simulink library "vmc"  (R2021b)
settings: Solver=VariableStepAuto  StartTime=0.0  StopTime=10.0  RelTol=1e-3
undefined symbols (not defined in the file or in its folder): AVMC_ACCDeltaTqIGain4OVRD_X_kph, AVMC_ACCDeltaTqIGain4OVRD_Y_mps2, AVMC_ACCDeltaTqIGain_X_kph, AVMC_ACCDeltaTqIGain_Y_mps2, AVMC_ACCDeltaTqPGain_X_kph, AVMC_ACCDeltaTqPGain_Y_kph, AVMC_ACCLongSteadyCtrl_X_kph, AVMC_ADSPosGFBDeltaTq_X_kph, AVMC_ADSPosGFBDeltaTq_Y_mps2, AVMC_AggressJerkPCT4AT_X_kph, AVMC_AggressJerkPCT_X_kph, AVMC_AggressLimitPCT4AT_X_kph, AVMC_AggressLimitPCT_X_kph, AVMC_CCLongSteadyCtrl_X_kph, AVMC_DISCDeltaTqIGain_X_kph, AVMC_DISCDeltaTqIGain_Y_mps2, AVMC_DISCDeltaTqPGain_X_kph, AVMC_DISCDeltaTqPGain_Y_kph, AVMC_ESCRegenOut_X_kph, AVMC_ESCRegenOut_Y_Deg, AVMC_ESCRegenOutEnSpd_X_Deg, AVMC_ISOAccLimit_X_mps, AVMC_ISODecLimit_X_mps, AVMC_ISOJerk_X_mps, AVMC_LatESCRegenOut_X_kph, AVMC_LatESCRegenOut_Y_Deg, AVMC_LongAccDeadZone_X_kph, AVMC_LongAccFiltTsforP2_X_Gps, AVMC_MCPresBaseTq_X_bar, AVMC_MSALongSteadyCtrl_X_kph, AVMC_MSAPedalOvrd_X_kph, AVMC_MSASpdBand_X_kph, AVMC_MSATqDownEndTq_X_kph, AVMC_MSATqDownTime_X_kph, AVMC_OPDDisSlideRate_X_Deg, AVMC_OVRD2ActSR2FCMCMD_X_mps2, AVMC_PedalTqRWhlRatio_X_Nm, AVMC_PedalTqRWhlRatio_Y_gps, AVMC_PedalTqRWhlSlipGain_X_rat, AVMC_PedalTqRWhlSlipGain_Y_kph, AVMC_PedalTqRWhSTRGGain_X_deg, AVMC_PedalTqRWhSTRGGain_Y_kph, AVMC_RDCDetectTime_X_kph, AVMC_RDCDetectTime_Y_pct, AVMC_RDCEnSlideRate_X_Deg, AVMC_RearWhlTqRatio_X_Nm, AVMC_RearWhlTqRatio_Y_gps, AVMC_RearWhlTqSlipGain_X_rat, AVMC_RearWhlTqSlipGain_Y_kph, AVMC_RearWhlTqSTRGGain_X_deg, AVMC_RearWhlTqSTRGGain_Y_kph, AVMC_ReqBrkJoinDecSR_X_mps2, AVMC_SoftJerkPCT_X_kph, AVMC_SoftLimitPCT_X_kph, AVMC_StESCYaw_X_kph, AVMC_StESCYaw_Y_Deg, AVMC_StESCYawCom_X_kph, AVMC_StESCYawCom_Y_Gps, AVMC_TMSpdBaseTq_X_rpm, AVMC_VehHoldDecCtrlTime2_X_kph ... (+411)
libraries: hcu_lib x108, simulink x82, tqr x1, simulink_extras x1
(part 7 of 14)

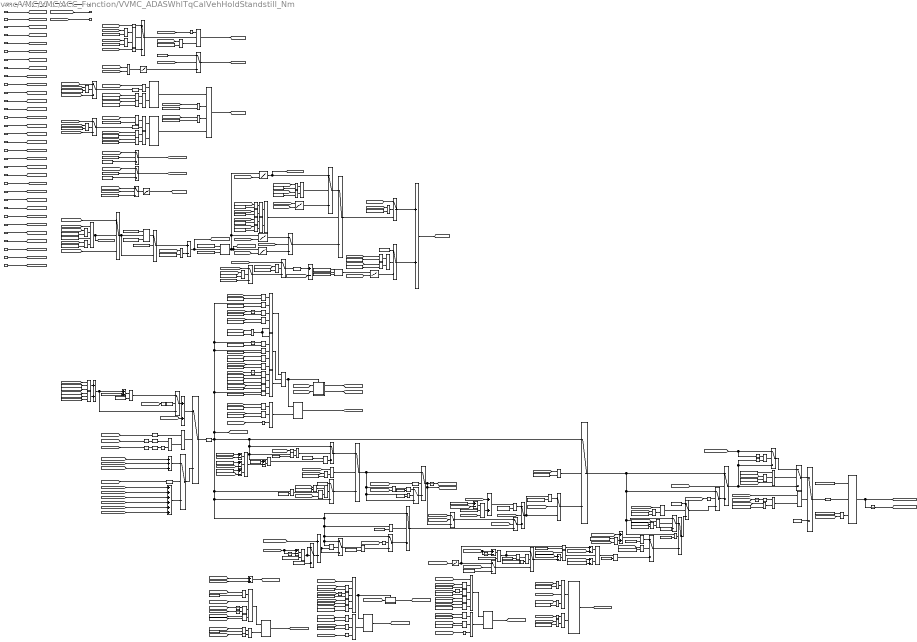
== system vmc/VMC/VMC/ACC_Function/VVMC_ADASWhlTqCalVehHoldStandstill_Nm ==
  note: Deceleration REGEN Torque Control
  note: Deceleration REGEN Torque Control Judgement
  note: Deceleration Torque Control
  note: Deceleration Positive Torque Control
  VVMC_LongAcc_Gps : Inport
  VVMC_ActACCRequiredAccel_mps2 : Inport  Port=2
  VINP_VehSpeed_kph : Inport  Port=3
  VVMC_ADASActive_flg : Inport  Port=4
  VTQD_CoordWhlTqDemFr_Nm : Inport  Port=5
  VTQD_CoordWhlTqDemRr_Nm : Inport  Port=6
  VVMC_ACCPedalOvrd_flg : Inport  Port=7
  VVMC_FeatSetSpdForCalcu_kph : Inport  Port=8
  VVMC_FeatArbitrFinal_enum : Inport  Port=9
  VINP_FrTMSpd_rpm : Inport  Port=10
  VINP_RrTMSpd_rpm : Inport  Port=11
  VINP_MCPressure_bar : Inport  Port=12
  VINP_ESCADASSta_enum : Inport  Port=13
  VVMC_FeatReqSpd_kph : Inport  Port=14
  VVMC_MeterIndSpeedForCalcu_kph : Inport  Port=15
  VTQD_SWC2ResUpSta_flg : Inport  Port=16
  VINP_FrntAxlTrqReqBrk_Nm : Inport  Port=17
  VINP_RearAxlTrqReqBrk_Nm : Inport  Port=18
  VTQR_RrTMTqReq_Nm : Inport  Port=19
  VVMC_ACCVehHoldReqRaw_flg : Inport  Port=20
  VVMC_EstSlope_Deg : Inport  Port=21
  VINP_TargetType_enum : Inport  Port=22
  VVMC_SafetyCtrl_flg : Inport  Port=23
  VTQR_FrTMTqReq_Nm : Inport  Port=24
  task_time_s : Inport  Port=25
  VVMC_TotalAvailBrkRgnTq_Nm : Inport  Port=26
  VVMC_AccelTurnHold_flg : Inport  Port=27
  VVMC_ADASACCSta_enum : Inport  Port=28
  VTQD_CreepBaseTqD_Nm : Inport  Port=29
  VVMC_OVRD2ActRampActive_flg : Inport  Port=30
  VINP_ACCRequiredAccel_mps2 : Inport  Port=31
  VTQD_SWC1ResUpSta_flg : Inport  Port=32
  VINP_SWCType_enum : Inport  Port=33
  " 1" : Constant  Value=ENUM_SWCTYPE_SWC2
  " 2" : Constant  Value=ENUM_SWCTYPE_SWC2
  AND{,1,4,7..8,10..11,13,17..18,20,29} (12 alike) : Logic  AllPortsSameDT=off  OutDataTypeStr=boolean
  AND12 : Logic  Inputs=3  AllPortsSameDT=off  OutDataTypeStr=boolean
  AND14 : Logic  Operator=OR  AllPortsSameDT=off  OutDataTypeStr=boolean
  AND19 : Logic  Operator=OR  AllPortsSameDT=off  OutDataTypeStr=boolean
  AND2 : Logic  Inputs=3  AllPortsSameDT=off  OutDataTypeStr=boolean
  AND3 : Logic  Inputs=4  AllPortsSameDT=off  OutDataTypeStr=boolean
  AND5 : Logic  Inputs=4  AllPortsSameDT=off  OutDataTypeStr=boolean
  AND6 : Logic  Inputs=3  AllPortsSameDT=off  OutDataTypeStr=boolean
  AND9 : Logic  Inputs=4  AllPortsSameDT=off  OutDataTypeStr=boolean
  Abs : Abs
  Abs1 : Abs
  Add{,3..4,7..8,10..12,14,16..17} (11 alike) : Sum  Inputs=+-
  Add1 : Sum  Inputs=++++++
  Add{2,5..6,13,15,19,21..23} (9 alike) : Sum
  Add9 : Sum  Inputs=+++
  Cast To Single2 : DataTypeConversion  OutDataTypeStr=single
  Cast To Single3 : DataTypeConversion  OutDataTypeStr=single
  Constant10 : Constant  Value=KVMC_ADASWhlTqUpperLim_Nm
  Constant100 : Constant  Value=KVMC_ZeroRgnTqSpdCtrlTime_s
  Constant{4,18..19,22,25,27,29,33,40,45,50..53,58,63..75,81..82,87,89..90,92..94,96,98..99,101..103,109,112,114,116..117,119..121,124..125,131..132,156,168} (56 alike) : Constant  Value=ZERO_FLOAT
  Constant104 : Constant  Value=KVMC_HoldAllowZeroTqGrade_deg
  Constant106 : Constant  Value=KVMC_VehHoldTqIncMinTq_Nm
  Constant107 : Constant  Value=KVMC_VehHoldTqIncMCP_bar
  Constant108 : Constant  Value=KVMC_VehHoldTqIncMCP_bar
  Constant11 : Constant  Value=KVMC_ADASWhlTqLowerLim_Nm
  Constant110 : Constant  Value=KVMC_NegReqEnSpd_kph
  Constant111 : Constant  Value=KVMC_VehHoldTqAlwaysIncSW_flg
  Constant12 : Constant  Value=KVMC_AccDevLowLim_mps2
  Constant122 : Constant  Value=KVMC_VehHoldDecSR_Nm
  Constant123 : Constant  Value=ENUM_FEATARBITRSTA_DISC
  Constant13 : Constant  Value=KVMC_AccDevUpLim_mps2
  Constant133 : Constant  Value=MINUSONE_FLOAT
  Constant138 : Constant  Value=KVMC_ReqAccelLimitSW_flg
  Constant139 : Constant  Value=KVMC_MaxReqAccel_mps2
  Constant14 : Constant  Value=KVMC_ACCSpdDevUpLim_kph
  Constant140 : Constant  Value=KVMC_MinReqAccel_mps2
  Constant15 : Constant  Value=KVMC_ACCSpdDevLowLim_kph
  Constant16 : Constant  Value=ENUM_FEATARBITRSTA_ACC
  Constant166 : Constant  Value=ENUM_ESCADASSTA_VEHASTANDSTILL
  Constant167 : Constant  Value=KVMC_StandstillTqRamp2ZeroSlope_Nmps
  Constant17 : Constant  Value=ENUM_ADASACCSTA_ACTIVE
  Constant{2,7..8,20} (4 alike) : Constant  Value=KVMC_HillUpResetTMSpd_rpm
  Constant21 : Constant  Value=ENUM_FEATARBITRSTA_DISC
  Constant23 : Constant  Value=KVMC_OVRDResSmoothTest_SW
  Constant24 : Constant  Value=KVMC_OVRD2ActRgnTarget_Nm
  Constant26 : Constant  Value=KVMC_AddBRegen2ACCLoop_flg
  Constant3 : Constant  Value=ENUM_ESCADASSTA_VEHASTANDSTILL
  Constant30 : Constant  Value=KVMC_TqSafetyCtrl_flg
  Constant31 : Constant  Value=KVMC_ACCResUpEnAccCMD_mps2
  Constant32 : Constant  Value=KVMC_TqMCPRelFactorHold_Nm
  Constant{6,36..37,62,77,80,88,97} (8 alike) : Constant  Value=KVMC_CutOffNegTqSpd_kph
  Constant38 : Constant  Value=KTQR_FrTMGearEff_c
  Constant{41,44,47..48,78..79,91} (7 alike) : Constant  Value=KVMC_ZeroRgnTqSpd_kph
  Constant42 : Constant  Value=KTQD_FrTMTotalGearRatio_gain
  Constant5 : Constant  Value=KVMC_AddBRegen2ACCLoop_flg
  Constant54 : Constant  Value=KVMC_NegReqSwEnSpd_kph
  Constant55 : Constant  Value=KVMC_NegReqSwEnSlope_Deg
  Constant56 : Constant  Value=KVMC_ACCResUpEnGrade_Deg
  Constant57 : Constant  Value=ENUM_TARGETTYPE_NONE
  Constant59 : Constant  Value=KVMC_TqMCPRelFactor_Nm
  Constant60 : Constant  Value=ENUM_FEATARBITRSTA_ACC
  Constant61 : Constant  Value=ENUM_FEATARBITRSTA_ACC
  Constant84 : Constant  Value=KTQD_RrTMTotalGearRatio_gain
  Constant85 : Constant  Value=KTQR_RrTMGearEff_c
  Constant86 : Constant  Value=KVMC_OVRDResTqDec4Smooth_Nm
  Constant9 : Constant  Value=KVMC_GravityValue_mps2
  Data Type Conversion1 : DataTypeConversion  OutDataTypeStr=single
  Detect Change : simulink/Logic and Bit Operations/Detect Change  vinit=0  OutDataTypeStr=boolean
  Detect Decrease1 : simulink/Logic and Bit Operations/Detect Decrease  vinit=0.0  OutDataTypeStr=boolean
  Detect Decrease2 : simulink/Logic and Bit Operations/Detect Decrease  vinit=0.0  OutDataTypeStr=boolean
  Detect Decrease3 : simulink/Logic and Bit Operations/Detect Decrease  vinit=0.0  OutDataTypeStr=boolean
  Detect Increase{1..4} (4 alike) : simulink/Logic and Bit Operations/Detect Increase  vinit=0.0  OutDataTypeStr=boolean
  Divide : Product  Inputs=*/*
  Divide1 : Product  Inputs=***
  Divide{2,4,7..8} (4 alike) : Product  Inputs=**
  Divide3 : Product  Inputs=*/*
  Divide5 : Product  Inputs=***
  Equal : RelationalOperator  Operator===  OutDataTypeStr=boolean  RndMeth=Simplest
  Equal1 : RelationalOperator  Operator=<=  OutDataTypeStr=boolean  RndMeth=Simplest
  Equal10 : RelationalOperator  Operator===  OutDataTypeStr=boolean  RndMeth=Simplest
  Equal{4,6,8,11} (4 alike) : RelationalOperator  Operator=<  OutDataTypeStr=boolean  RndMeth=Simplest
  Equal12 : RelationalOperator  Operator=>  OutDataTypeStr=boolean  RndMeth=Simplest
  Equal2 : RelationalOperator  Operator=~=  OutDataTypeStr=boolean  RndMeth=Simplest
  Equal3 : RelationalOperator  OutDataTypeStr=boolean  RndMeth=Simplest
  Equal5 : RelationalOperator  OutDataTypeStr=boolean  RndMeth=Simplest
  Equal7 : RelationalOperator  Operator=>  OutDataTypeStr=boolean  RndMeth=Simplest
  Equal9 : RelationalOperator  Operator=>  OutDataTypeStr=boolean  RndMeth=Simplest
  InitialCondition: 1 : UnitDelay  SampleTime=-1  HasFrameUpgradeWarning=on
  Logical Operator : Logic  Inputs=4  AllPortsSameDT=off  OutDataTypeStr=boolean
  Logical Operator1 : Logic  Operator=OR  AllPortsSameDT=off  OutDataTypeStr=boolean
  Logical Operator{2,4,6,8} (4 alike) : Logic  Inputs=5  AllPortsSameDT=off  OutDataTypeStr=boolean
  Logical Operator3 : Logic  Operator=OR  Inputs=3  AllPortsSameDT=off  OutDataTypeStr=boolean
  Logical Operator5 : Logic  AllPortsSameDT=off  OutDataTypeStr=boolean
  Logical Operator7 : Logic  Operator=OR  Inputs=3  AllPortsSameDT=off  OutDataTypeStr=boolean
  Logical Operator9 : Logic  Operator=OR  Inputs=3  AllPortsSameDT=off  OutDataTypeStr=boolean
  MVMC_ACCDeltaTqIGain4OVRD_Z_Nm : Lookup_n-D  BreakpointsForDimension1=AVMC_ACCDeltaTqIGain4OVRD_Y_mps2  BreakpointsForDimension2=AVMC_ACCDeltaTqIGain4OVRD_X_kph  Table=MVMC_ACCDeltaTqIGain4OVRD_Z_Nm  InternalRulePriority=Speed  RndMeth=Simplest  InputSameDT=on
      settings: InputPortMap=u0,u1
  MVMC_ACCDeltaTqIGain_Z_Nm : Lookup_n-D  BreakpointsForDimension1=AVMC_ACCDeltaTqIGain_Y_mps2  BreakpointsForDimension2=AVMC_ACCDeltaTqIGain_X_kph  Table=MVMC_ACCDeltaTqIGain_Z_Nm  InternalRulePriority=Speed  RndMeth=Simplest  InputSameDT=on
      settings: InputPortMap=u0,u1
  MVMC_ACCDeltaTqPGain_Z_Nm1 : Lookup_n-D  BreakpointsForDimension1=AVMC_ACCDeltaTqPGain_Y_kph  BreakpointsForDimension2=AVMC_ACCDeltaTqPGain_X_kph  Table=MVMC_ACCDeltaTqPGain_Z_Nm  InternalRulePriority=Speed  RndMeth=Simplest  InputSameDT=on
      settings: InputPortMap=u0,u1
  MVMC_ADSPosGFBDeltaTq_Z_Nm1 : Lookup_n-D  BreakpointsForDimension1=AVMC_ADSPosGFBDeltaTq_Y_mps2  BreakpointsForDimension2=AVMC_ADSPosGFBDeltaTq_X_kph  Table=MVMC_ADSPosGFBDeltaTq_Z_Nm  InternalRulePriority=Speed  RndMeth=Simplest  InputSameDT=on
      settings: InputPortMap=u0,u1
  MVMC_DISCDeltaTqIGain_Z_Nm : Lookup_n-D  BreakpointsForDimension1=AVMC_DISCDeltaTqIGain_Y_mps2  BreakpointsForDimension2=AVMC_DISCDeltaTqIGain_X_kph  Table=MVMC_DISCDeltaTqIGain_Z_Nm  InternalRulePriority=Speed  RndMeth=Simplest  InputSameDT=on
      settings: InputPortMap=u0,u1
  MVMC_MCPresBaseTq_Y_Nm : Lookup_n-D  NumberOfTableDimensions=1  BreakpointsForDimension1=AVMC_MCPresBaseTq_X_bar  Table=MVMC_MCPresBaseTq_Y_Nm  InternalRulePriority=Speed  RndMeth=Simplest  InputSameDT=on
  MVMC_TMSpdBaseTq_Y_Nm : Lookup_n-D  NumberOfTableDimensions=1  BreakpointsForDimension1=AVMC_TMSpdBaseTq_X_rpm  Table=MVMC_TMSpdBaseTq_Y_Nm  InternalRulePriority=Speed  RndMeth=Simplest  InputSameDT=on
  MVMC_VehHoldTqIncGain_Y_Nm : Lookup_n-D  NumberOfTableDimensions=1  BreakpointsForDimension1=AVMC_VehHoldTqIncGain_X_deg  Table=MVMC_VehHoldTqIncGain_Y_Nm  InternalRulePriority=Speed  RndMeth=Simplest  InputSameDT=on
  Max{,1,4..6,8} (6 alike) : MinMax  Function=max  Inputs=2
  Max2 : MinMax  Inputs=2
  Max3 : MinMax  Inputs=2
  Max9 : MinMax  Inputs=2
  Min : MinMax  Inputs=2
  Min1 : MinMax  Inputs=2
  Min2 : MinMax  Function=max  Inputs=2
  Min5 : MinMax  Function=max  Inputs=2
  NOT{,1..10,13} (12 alike) : Logic  Operator=NOT  AllPortsSameDT=off  OutDataTypeStr=boolean
  OR{,1,4,6..8} (6 alike) : Logic  Operator=OR  AllPortsSameDT=off  OutDataTypeStr=boolean
  OR3 : Logic  Operator=OR  Inputs=3  AllPortsSameDT=off  OutDataTypeStr=boolean
  OR5 : Logic  AllPortsSameDT=off  OutDataTypeStr=boolean
  Product1 : Product
  Relational Operator{,2..4,7,13,16,27,32..33,38,44,47,58..59,61} (16 alike) : RelationalOperator  Operator=>  OutDataTypeStr=boolean  RndMeth=Simplest
  Relational Operator{1,18,20,34,40,51} (6 alike) : RelationalOperator  Operator=<=  OutDataTypeStr=boolean  RndMeth=Simplest
  Relational Operator{8,10,12,24..25,29,36..37,39,42..43,48,53} (13 alike) : RelationalOperator  OutDataTypeStr=boolean  RndMeth=Simplest
  Relational Operator{9,11,14..15,21..23,26,28,30..31,35,41,45..46,49..50,52,54} (19 alike) : RelationalOperator  Operator=<  OutDataTypeStr=boolean  RndMeth=Simplest
  Relational Operator{5..6,17,19,55..57,73} (8 alike) : RelationalOperator  Operator===  OutDataTypeStr=boolean  RndMeth=Simplest
  Relay : Relay  OnSwitchValue=KVMC_ACCTq2ZeroEnMCPress2_bar  OffSwitchValue=KVMC_ACCTq2ZeroDisMCPress2_bar  OutDataTypeStr=boolean
  Relay1 : Relay  OnSwitchValue=KVMC_ACCTq2ZeroEnMCPress_bar  OffSwitchValue=KVMC_ACCTq2ZeroDisMCPress_bar  OutDataTypeStr=boolean
  SR_Latch{,1..6} (7 alike) : hcu_lib/Basic_Blocks/SR_Latch
  Saturation Dynamic{1..5} (5 alike) : simulink/Discontinuities/Saturation Dynamic  OutMin=[]  OutMax=[]  OutDataTypeStr=Inherit: Same as second input  OutDataType=fixdt(1, 16)  OutScaling=2^-10  DoSatur=off
  Switch{,1..34,36..37,39..41} (40 alike) : Switch  Criteria=u2 > Threshold
  Triggered Subsystem1 : Subsystem  TreatAsAtomicUnit=on
  Triggered Subsystem4 : Subsystem  TreatAsAtomicUnit=on
  Unit Delay{,1..13} (14 alike) : UnitDelay  SampleTime=-1  HasFrameUpgradeWarning=on
  u2 > 0 : Switch  Criteria=u2 > Threshold
  u2 > 0 (1) : Switch  Criteria=u2 > Threshold
  u2 > 0 (3) : Switch  Criteria=u2 > Threshold
  u2 > 0 (4) : Switch  Criteria=u2 > Threshold
  VVMC_ADASWhlTqCal_Nm : Outport
  VVMC_ADASNegReq_flg : Outport  Port=2
  VVMC_ACCLowSpdTqCtrl_flg : Outport  Port=3
  wires:
  VVMC_FeatReqSpd_kph/1 -> [VVMC_FeatReqSpd_kph]
  [VINP_RrTMSpd_rpm] -> Relational Operator2/1
  [VVMC_ACCVehHoldReqRaw_flg] -> AND4/1
  MVMC_MCPresBaseTq_Y_Nm/1 -> [VVMC_MCPresBaseTq_Nm]  "VVMC_MCPresBaseTq_Nm"
  Switch1/1 -> MVMC_MCPresBaseTq_Y_Nm/1
  [VINP_MCPressure_bar] -> Switch1/1
  Relational Operator/1 -> OR/1
  Equal/1 -> AND1/1
  OR/1 -> SR_Latch/2
  [VINP_FrTMSpd_rpm] -> Relational Operator/1
  [VINP_ESCADASSta_enum] -> Equal/1
  [VINP_RrTMSpd_rpm] -> Relational Operator4/1
  AND1/1 -> SR_Latch1/1
  Relational Operator2/1 -> OR/2
  OR1/1 -> SR_Latch1/2
  Constant19/1 -> Switch1/3
  Constant8/1 -> Relational Operator3/2
  Relational Operator4/1 -> OR1/2
  [VVMC_MCPreBaseTqEn_flg] -> Switch1/2
  [VINP_FrTMSpd_rpm] -> Relational Operator3/1
  Constant7/1 -> Relational Operator4/2
  Constant2/1 -> Relational Operator2/2
  Detect Increase3/1 -> AND1/2
  SR_Latch/1 -> AND3/1  "VVMC_HillUpHoldReqEn_flg"
  AND3/1 -> [VVMC_MCPreBaseTqEn_flg]  "VVMC_MCPreBaseTqEn_flg"
  SR_Latch1/1 -> AND3/4  "VVMC_HillUpESCStaEn_flg"
  Constant3/1 -> Equal/2
  Constant20/1 -> Relational Operator/2
  Relational Operator3/1 -> OR1/1
  VINP_FrTMSpd_rpm/1 -> [VINP_FrTMSpd_rpm]
  VINP_RrTMSpd_rpm/1 -> [VINP_RrTMSpd_rpm]
  VINP_MCPressure_bar/1 -> [VINP_MCPressure_bar]
  VINP_ESCADASSta_enum/1 -> [VINP_ESCADASSta_enum]
  VVMC_FeatArbitrFinal_enum/1 -> [VVMC_FeatArbitrFinal_enum]
  VVMC_LongAcc_Gps/1 -> [VVMC_LongAcc_Gps]
  VVMC_ActACCRequiredAccel_mps2/1 -> [VVMC_ActACCRequiredAccel_mps2]
  VINP_VehSpeed_kph/1 -> [VINP_VehSpeed_kph]
  VVMC_ADASActive_flg/1 -> [VVMC_ADASActive_flg]
  [VVMC_ADASWhlTqCal_Nm] -> VVMC_ADASWhlTqCal_Nm/1
  VTQD_CoordWhlTqDemFr_Nm/1 -> [VTQD_CoordWhlTqDemFr_Nm]
  VTQD_CoordWhlTqDemRr_Nm/1 -> [VTQD_CoordWhlTqDemRr_Nm]
  VVMC_ACCPedalOvrd_flg/1 -> [VVMC_ACCPedalOvrd_flg]
  VVMC_FeatSetSpdForCalcu_kph/1 -> [VVMC_FeatSetSpdForCalcu_kph]
  VINP_RearAxlTrqReqBrk_Nm/1 -> [VINP_RearAxlTrqReqBrk_Nm]
  VINP_FrntAxlTrqReqBrk_Nm/1 -> [VINP_FrntAxlTrqReqBrk_Nm]
  VTQD_SWC2ResUpSta_flg/1 -> [VTQD_SWC2ResUpSta_flg]
  VVMC_MeterIndSpeedForCalcu_kph/1 -> [VVMC_MeterIndSpeedForCalcu_kph]
  Switch32/1 -> Detect Increase2/1
  AND4/1 -> SR_Latch/1
  [VVMC_ActACCRequiredAccel_mps2] -> Relational Operator7/1
  Constant31/1 -> Relational Operator7/2
  Switch2/1 -> Detect Increase3/1
  [VINP_FrntAxlTrqReqBrk_Nm] -> Switch3/1
  [VINP_RearAxlTrqReqBrk_Nm] -> Switch4/1
  Constant25/1 -> Switch3/3
  Constant27/1 -> Switch4/3
  Constant26/1 -> Switch4/2
  Switch4/1 -> [VVMC_RearAxlTrqReqBrk_Nm]  "VVMC_RearAxlTrqReqBrk_Nm"
  Switch3/1 -> [VVMC_FrntAxlTrqReqBrk_Nm]  "VVMC_FrntAxlTrqReqBrk_Nm"
  Constant5/1 -> Switch3/2
  [VVMC_ADASNegReq_flg] -> VVMC_ADASNegReq_flg/1
  VTQR_RrTMTqReq_Nm/1 -> [VTQR_RrTMTqReq_Nm]
  VVMC_ACCVehHoldReqRaw_flg/1 -> [VVMC_ACCVehHoldReqRaw_flg]
  [VVMC_EstSlope_Deg] -> Relational Operator16/1
  Relational Operator16/1 -> AND3/3
  Constant56/1 -> Relational Operator16/2
  VVMC_EstSlope_Deg/1 -> [VVMC_EstSlope_Deg]
  VINP_TargetType_enum/1 -> [VINP_TargetType_enum]
  VVMC_SafetyCtrl_flg/1 -> [VVMC_SafetyCtrl_flg]
  VTQR_FrTMTqReq_Nm/1 -> [VTQR_FrTMTqReq_Nm]
  [VVMC_ACCLowSpdTqCtrl_flg] -> VVMC_ACCLowSpdTqCtrl_flg/1
  task_time_s/1 -> [task_time_s]
  MVMC_TMSpdBaseTq_Y_Nm/1 -> Switch/3
  [VVMC_ACCVehHoldReqRaw_flg] -> Switch/2
  Relay/1 -> Switch13/1
  Switch13/1 -> AND2/2  "VVMC_ADASNegReqAct_flg"
  AND2/1 -> [VVMC_ADASNegReq_flg]  "VVMC_ADASNegReq_flg"
  [VINP_RrTMSpd_rpm] -> Min/2
  [VVMC_MCPreBaseTqEn_flg] -> NOT2/1
  Equal5/1 -> AND2/3
  [VINP_VehSpeed_kph] -> Equal5/1
  [VINP_FrTMSpd_rpm] -> Min/1
  Constant110/1 -> Equal5/2
  [VINP_MCPressure_bar] -> Relay/1
  [VINP_VehSpeed_kph] -> Equal1/1
  Equal3/1 -> AND10/2
  Relay1/1 -> Switch13/3
  Switch/1 -> [VVMC_TMSpdBaseTq_Nm]  "VVMC_TMSpdBaseTq_Nm"
  Constant54/1 -> Equal1/2
  [VINP_MCPressure_bar] -> Relay1/1
  AND10/1 -> Switch13/2
  Constant55/1 -> Equal3/2
  [VVMC_EstSlope_Deg] -> Equal3/1
  Equal1/1 -> AND10/1
  Min/1 -> MVMC_TMSpdBaseTq_Y_Nm/1
  NOT2/1 -> AND2/1
  Constant119/1 -> Switch/1
  Switch29/1 -> Switch22/3
  [VINP_VehSpeed_kph] -> Relational Operator21/1
  [VINP_VehSpeed_kph] -> Relational Operator20/1
  Relational Operator11/1 -> Logical Operator/2
  SR_Latch4/1 -> [VVMC_ZeroRgnTqSpdCtrl_flg]  "VVMC_ZeroRgnTqSpdCtrl_flg"
  Constant48/1 -> Add4/1
  Relational Operator31/1 -> Logical Operator4/1
  [VVMC_ActACCRequiredAccel_mps2] -> Relational Operator41/1
  Logical Operator2/1 -> OR3/2
  Constant93/1 -> Relational Operator42/2
  Relational Operator25/1 -> Logical Operator2/2
  Max1/1 -> Switch23/1
  Logical Operator/1 -> OR3/3
  [VVMC_LastADASWhlTqCal_Nm] -> Add12/1
  [VINP_VehSpeed_kph] -> Relational Operator8/1
  [VVMC_ADASActive_flg] -> NOT1/1
  Constant63/1 -> Min2/2
  Logical Operator3/1 -> SR_Latch6/2
  Constant29/1 -> Relational Operator10/2
  Relational Operator8/1 -> Logical Operator3/1
  Unit Delay/1 -> Relational Operator12/1
  [VVMC_TMSpdBaseTq_Nm] -> Add1/3
  Logical Operator1/1 -> Switch6/2
  Constant36/1 -> Relational Operator11/2
  NOT1/1 -> Logical Operator3/3
  [VINP_MCPressure_bar] -> Add11/1, Unit Delay5/1
  [VVMC_FrntAxlTrqReqBrk_Nm] -> Add1/5
  [VTQD_CoordWhlTqDemFr_Nm] -> Add9/1
  Divide2/1 -> Switch15/1, Switch15/2
  Constant92/1 -> Relational Operator41/2
  Constant84/1 -> Divide5/2
  Relational Operator15/1 -> Logical Operator/4
  [VVMC_ActACCRequiredAccel_mps2] -> Relational Operator10/1
  Constant114/1 -> Relational Operator49/2
  AND13/1 -> Switch21/2
  Constant69/1 -> Switch15/3
  Add14/1 -> Divide3/1
  Constant101/1 -> Max2/2
  Switch23/1 -> Switch17/3  "VVMC_ADASWhlTqCalNegCMD_Nm"
  Constant70/1 -> Relational Operator26/2
  [VVMC_MCPresBaseTq_Nm] -> Add1/4
  [VINP_VehSpeed_kph] -> Relational Operator44/1
  Switch10/1 -> Min2/1
  Constant64/1 -> Relational Operator22/2
  Min2/1 -> Switch16/3  "VVMC_ACCTqNegReq_Nm"
  [VTQR_RrTMTqReq_Nm] -> Divide5/1
  Triggered Subsystem1/2(Out2) -> [VVMC_ACCLowSpdCtrlEnSpd_kph]  "VVMC_ACCLowSpdCtrlEnSpd_kph"
  NOT9/1 -> Logical Operator9/3
  Switch6/1 -> Cast To Single2/1
  Logical Operator8/1 -> SR_Latch4/1, Triggered Subsystem4/Trigger
  Cast To Single2/1 -> Switch19/1, Relational Operator26/1, Switch16/1, Switch10/1, Relational Operator9/1, Switch21/3, Relational Operator49/1, Switch27/1, Max4/1, Relational Operator47/1, Switch17/1, [VVMC_OriADASWhlTq_Nm], Relational Operator30/1, Unit Delay3/1, Relational Operator23/1, Relational Operator15/1  "VVMC_OriADASWhlTq_Nm"
  Add11/1 -> Divide2/1
  Unit Delay7/1 -> [VVMC_LastACCLowSpdTq_Nm]
  Detect Increase1/1 -> Logical Operator1/1
  [VVMC_ZeroRgnTqSpdCtrl_flg] -> Switch24/2
  Add15/1 -> Max2/1  "VVMC_ADASWhlTqCalZeroRgnCtrl_Nm"
  Add5/1 -> Switch6/1
  Divide1/1 -> Add13/1
  Triggered Subsystem4/1(Out1) -> [VVMC_ZeroRgnTqSpdCtrlTq_Nm]  "VVMC_ZeroRgnTqSpdCtrlTq_Nm"
  Unit Delay9/1 -> Relational Operator42/1
  Detect Decrease2/1 -> Switch8/2
  Add13/1 -> Switch36/3, Add23/1
  [VVMC_LastADASWhlTqCal_Nm] -> Relational Operator45/1
  Relational Operator32/1 -> Logical Operator4/5, Logical Operator2/1
  [VVMC_LastADASWhlTqCal_Nm] -> Triggered Subsystem4/1(In1)
  Constant96/1 -> Relational Operator43/2
  [VINP_VehSpeed_kph] -> Relational Operator40/1
  Divide/1 -> Add/2
  Constant67/1 -> Relational Operator25/2
  Relational Operator44/1 -> Logical Operator9/1
  Relational Operator30/1 -> Logical Operator4/2
  Switch21/1 -> Switch12/3  "VVMC_ACCLowSpdTqEnSpdLo_Nm"
  [VVMC_ActACCRequiredAccel_mps2] -> Unit Delay6/1
  [VVMC_ActACCRequiredAccel_mps2] -> Relational Operator43/1
  Constant97/1 -> Relational Operator44/2
  [VVMC_ADASActive_flg] -> NOT9/1
  Add/1 -> Max4/2
  Relational Operator29/1 -> Logical Operator4/3
  Relational Operator45/1 -> Logical Operator8/2
  Constant98/1 -> Relational Operator45/2
  Constant6/1 -> Relational Operator8/2
  [VVMC_ActACCRequiredAccel_mps2] -> Unit Delay9/1
  Switch18/1 -> Switch24/3
  Add1/1 -> Switch8/3
  Constant100/1 -> Divide3/2
  Constant89/1 -> Max1/2
  [VVMC_RgnProhibited_flg] -> Switch23/2
  [VINP_VehSpeed_kph] -> Relational Operator31/1
  [task_time_s] -> Divide3/3
  Constant53/1 -> Switch21/1
  Max2/1 -> Switch24/1
  Constant99/1 -> Add14/1
  Relational Operator12/1 -> Logical Operator/1
  [VVMC_LastACCLowSpdTq_Nm] -> Max/2
  Switch12/1 -> Switch22/1, Switch29/3, Relational Operator50/1, Max/1
  Switch15/1 -> Add12/2
  Constant117/1 -> Max3/2
  Add9/1 -> Switch8/1
  [VVMC_ActACCRequiredAccel_mps2] -> Relational Operator24/1
  [VVMC_ACCLowSpdCtrlEnSpd_kph] -> Add4/2
  Min1/1 -> Switch27/3
  Relational Operator20/1 -> AND13/1
  Relational Operator47/1 -> AND8/2
  Max/1 -> Max3/1
  Relational Operator43/1 -> Logical Operator9/2
  Constant47/1 -> Add3/1
  [VVMC_ACCLowSpdTqCtrl_flg] -> Detect Increase4/1
  Constant4/1 -> Relational Operator24/2
  Unit Delay5/1 -> Add11/2
  Max3/1 -> Switch29/1
  Detect Increase4/1 -> Switch22/2
  Constant78/1 -> Relational Operator32/2
  Constant79/1 -> Relational Operator33/2
  [VINP_VehSpeed_kph] -> Relational Operator32/1
  [VVMC_ACCLowSpdCtrlEnSpd_kph] -> Relational Operator33/1
  [VVMC_ZeroRgnTqSpdCtrlTq_Nm] -> Add14/2
  Constant77/1 -> Relational Operator31/2
  Constant75/1 -> Relational Operator30/2
  Logical Operator4/1 -> OR3/1
  Constant73/1 -> Relational Operator29/2
  Relational Operator42/1 -> Logical Operator8/3
  Constant72/1 -> Relational Operator28/2
  [VVMC_ADASActive_flg] -> Detect Increase1/1
  Relational Operator28/1 -> Logical Operator4/4
  [VVMC_ActACCRequiredAccel_mps2] -> Relational Operator28/1
  [VVMC_RearAxlTrqReqBrk_Nm] -> Add1/6
  Constant40/1 -> Relational Operator14/2
  Relational Operator41/1 -> Logical Operator8/4
  Switch24/1 -> Max1/1, Switch23/3
  [VINP_VehSpeed_kph] -> Unit Delay/1
  [VINP_VehSpeed_kph] -> Triggered Subsystem1/2(In2)
  Unit Delay3/1 -> Relational Operator25/1
  Relational Operator26/1 -> Switch19/2
  AND14/1 -> AND13/2
  Constant38/1 -> Divide1/3
  Switch22/1 -> Unit Delay7/1, Switch20/3, [VVMC_ACCLowSpdTq_Nm]  "VVMC_ACCLowSpdTq_Nm"
  [VVMC_ACCLowSpdTqCtrl_flg] -> Logical Operator5/1
  OR3/1 -> SR_Latch6/1, Triggered Subsystem1/Trigger
  Relational Operator23/1 -> Logical Operator2/3
  [VVMC_ActACCRequiredAccel_mps2] -> Relational Operator22/1
  [VTQR_FrTMTqReq_Nm] -> Divide1/1
  Switch27/1 -> Switch12/1  "VVMC_ACCLowSpdTqEnSpdHi_Nm"
  Relational Operator21/1 -> Logical Operator2/4
  Constant62/1 -> Relational Operator21/2
  Relational Operator10/1 -> Logical Operator3/2
  Unit Delay6/1 -> Relational Operator29/1
  [VINP_VehSpeed_kph] -> Relational Operator11/1
  Add10/1 -> Divide/3
  Constant112/1 -> Relational Operator47/2
  Logical Operator5/1 -> Switch12/2
  AND/1 -> Logical Operator1/2
  Constant52/1 -> Min1/1
  Relational Operator9/1 -> Switch10/2
  Add12/1 -> Relational Operator9/2, Switch10/3  "VVMC_ACCTqRampOutByMCP_Nm"
  Add4/1 -> Divide/2
  [VVMC_LastADASWhlTqCal_Nm] -> Add15/1
  Add3/1 -> Divide/1
  [VVMC_ADASNegReq_flg] -> Detect Decrease2/1
  Divide5/1 -> Add13/2
  Relational Operator24/1 -> Switch17/2
  Constant85/1 -> Divide5/3
  Constant50/1 -> Add10/1
  Constant37/1 -> Relational Operator12/2
  [VVMC_ACCDeltaTq_Nm] -> Add9/3
  Relational Operator22/1 -> Logical Operator2/5
  Constant66/1 -> Relational Operator23/2
  Constant45/1 -> Relational Operator15/2
  Relational Operator40/1 -> Logical Operator8/5
  Constant42/1 -> Divide1/2
  [VVMC_ActACCRequiredAccel_mps2] -> Relational Operator14/1
  Relational Operator14/1 -> Logical Operator/3
  [VVMC_ACCDeltaTq_Nm] -> Add1/2
  [VVMC_LastADASWhlTqCal_Nm] -> Add1/1
  [VVMC_ACCLowSpdTqLimit_Nm] -> Add10/2
  Triggered Subsystem1/1(Out1) -> [VVMC_ACCLowSpdTqLimit_Nm]  "VVMC_ACCLowSpdTqLimit_Nm"
  Constant116/1 -> Relational Operator50/2
  Relational Operator33/1 -> Logical Operator5/2
  [VINP_VehSpeed_kph] -> Add3/2
  Constant51/1 -> Add/1
  [VVMC_ACCLowSpdTqCtrl_flg] -> Switch18/2
  [VTQD_CoordWhlTqDemRr_Nm] -> Add9/2
  SR_Latch6/1 -> [VVMC_ACCLowSpdTqCtrl_flg]  "VVMC_ACCLowSpdTqCtrl_flg"
  Constant91/1 -> Relational Operator40/2
  Constant41/1 -> Relational Operator20/2
  Divide3/1 -> Add15/2
  [VVMC_ACCDeltaTq_Nm] -> Add5/2
  Constant59/1 -> Divide2/2
  Relational Operator49/1 -> AND14/1
  AND8/1 -> Switch27/2
  NOT13/1 -> AND8/1
  [VVMC_ADASNegReq_flg] -> NOT13/1
  Constant12/1 -> Saturation Dynamic4/3
  Saturation Dynamic4/1 -> MVMC_DISCDeltaTqIGain_Z_Nm/1, MVMC_ACCDeltaTqIGain4OVRD_Z_Nm/1, [VVMC_ActAccDev_mps2], MVMC_ACCDeltaTqIGain_Z_Nm/1  "VVMC_ActAccDev_mps2"
  Switch33/1 -> Add6/1  "VVMC_ACCDeltaTqIGain_Nm"
  Saturation Dynamic5/1 -> MVMC_ACCDeltaTqPGain_Z_Nm1/1  "VVMC_ACCActSpdDev_kph"
  [VVMC_LongAcc_Gps] -> Product1/1
  Constant16/1 -> Relational Operator5/2
  [VVMC_FeatArbitrFinal_enum] -> Relational Operator6/1
  [VVMC_FeatArbitrFinal_enum] -> Relational Operator5/1
  [VVMC_FeatReqSpd_kph] -> u2 > 0 (1)/1
  Constant15/1 -> Saturation Dynamic5/3
  Equal2/1 -> AND11/1
  Product1/1 -> Add7/2
  Constant21/1 -> Relational Operator6/2
  Constant60/1 -> Relational Operator17/2
  u2 > 0/1 -> Data Type Conversion1/1
  u2 > 0 (1)/1 -> u2 > 0/3
  [VVMC_MeterIndSpeedForCalcu_kph] -> Add8/2
  [VVMC_LongAcc_Gps] -> Equal6/1
  AND17/1 -> AND19/1
  [VVMC_ActACCRequiredAccel_mps2] -> Equal7/1
  [VINP_VehSpeed_kph] -> MVMC_DISCDeltaTqIGain_Z_Nm/2
  Constant125/1 -> Equal7/2
  [VINP_TargetType_enum] -> Equal2/1
  MVMC_DISCDeltaTqIGain_Z_Nm/1 -> [VVMC_DISCDeltaTqIGain_Nm], Switch40/1  "VVMC_DISCDeltaTqIGain_Nm"
  Constant124/1 -> Equal6/2
  Data Type Conversion1/1 -> Add8/1
  Relational Operator5/1 -> u2 > 0/2
  Add6/1 -> [VVMC_ACCDeltaTq_Nm]  "VVMC_ACCDeltaTq_Nm"
  MVMC_ACCDeltaTqIGain_Z_Nm/1 -> Switch26/3  "VVMC_ACCDeltaTqIGainOri_Nm"
  Constant13/1 -> Saturation Dynamic4/1
  [VVMC_FeatArbitrFinal_enum] -> Relational Operator55/1
  Relational Operator55/1 -> Switch33/2
  Constant9/1 -> Product1/2
  [VINP_VehSpeed_kph] -> MVMC_ACCDeltaTqIGain_Z_Nm/2
  Equal6/1 -> AND17/1
  Add8/1 -> Saturation Dynamic5/2
  [VINP_VehSpeed_kph] -> MVMC_ACCDeltaTqPGain_Z_Nm1/2
  Add7/1 -> [VVMC_ACCDeltaAccel_mps2], Saturation Dynamic4/2  "VVMC_ACCDeltaAccel_mps2"
  Constant123/1 -> Relational Operator55/2
  Constant22/1 -> u2 > 0 (1)/3
  Constant14/1 -> Saturation Dynamic5/1
  Equal7/1 -> AND17/2
  AND11/1 -> Switch14/2
  Relational Operator6/1 -> u2 > 0 (1)/2
  [VVMC_FeatSetSpdForCalcu_kph] -> u2 > 0/1
  MVMC_ACCDeltaTqPGain_Z_Nm1/1 -> Switch14/3
  Relational Operator17/1 -> AND11/2
  [VVMC_FeatArbitrFinal_enum] -> Relational Operator17/1
  Constant57/1 -> Equal2/2
  Switch34/1 -> Switch33/3
  Constant58/1 -> Switch14/1
  Switch14/1 -> Add6/2  "VVMC_ACCDeltaTqPGain_Nm"
  AND19/1 -> Switch34/2
  Constant131/1 -> Equal8/2
  [VVMC_ActACCRequiredAccel_mps2] -> Equal8/1
  Equal8/1 -> AND20/1
  AND20/1 -> AND19/2
  Equal9/1 -> AND20/2
  [VVMC_ACCDeltaAccel_mps2] -> Equal9/1
  Constant132/1 -> Equal9/2
  Switch19/1 -> Switch18/3  "VVMC_ACCTqNegReqNotLowSpd_Nm"
  Detect Increase2/1 -> AND4/2
  Relational Operator7/1 -> AND3/2
  VVMC_TotalAvailBrkRgnTq_Nm/1 -> [VVMC_TotalAvailBrkRgnTq_Nm]
  VVMC_AccelTurnHold_flg/1 -> [VVMC_AccelTurnHold_flg]
  VVMC_ADASACCSta_enum/1 -> [VVMC_ADASACCSta_enum]
  Unit Delay1/1 -> Detect Decrease3/1
  Detect Change/1 -> NOT/1
  NOT/1 -> AND/2
  [VVMC_ACCPedalOvrd_flg] -> Unit Delay1/1
  [VVMC_FeatArbitrFinal_enum] -> Unit Delay2/1
  Unit Delay2/1 -> Detect Change/1
  Detect Decrease3/1 -> AND/1
  Switch8/1 -> Switch6/3
  Saturation Dynamic1/1 -> Switch37/1
  Constant139/1 -> Saturation Dynamic1/1
  Switch9/1 -> Switch37/3, Saturation Dynamic1/2
  Constant140/1 -> Saturation Dynamic1/3
  Constant138/1 -> Switch37/2
  Switch37/1 -> Add7/1
  [VVMC_ADASNegReq_flg] -> NOT5/1
  Switch16/1 -> Switch19/3
  NOT5/1 -> Switch16/2
  [VVMC_ADASNegReq_flg] -> AND14/2
  [VINP_RearAxlTrqReqBrk_Nm] -> Add2/2
  [VINP_FrntAxlTrqReqBrk_Nm] -> Add2/1
  Add2/1 -> [VVMC_TotalESCBRgnReq_Nm]
  [VVMC_ACCLowSpdTq_Nm] -> Unit Delay10/1
  Unit Delay10/1 -> Relational Operator46/1
  [VVMC_TotalESCBRgnReq_Nm] -> Unit Delay11/1
  Unit Delay11/1 -> Relational Operator46/2
  [VVMC_TotalESCBRgnReq_Nm] -> Relational Operator48/2
  [VVMC_ACCLowSpdTq_Nm] -> Relational Operator48/1
  Relational Operator46/1 -> AND5/3
  Relational Operator48/1 -> AND5/4
  AND5/1 -> SR_Latch5/1
  [VVMC_ACCLowSpdTqCtrl_flg] -> AND5/2
  SR_Latch5/1 -> [VVMC_ACCLowSpdFollowESCTq_flg]  "VVMC_ACCLowSpdFollowESCTq_flg"
  Max4/1 -> Min1/2
  [VVMC_TotalESCBRgnReq_Nm] -> Switch20/1
  [VVMC_ACCLowSpdFollowESCTq_flg] -> Switch20/2
  Relational Operator50/1 -> Switch29/2
  Switch20/1 -> Switch18/1  "VVMC_ACCLowSpdTqAftFollowESC_Nm"
  VTQD_CreepBaseTqD_Nm/1 -> [VTQD_CreepBaseTqD_Nm]
  Constant109/1 -> Relational Operator58/2
  Relational Operator58/1 -> OR7/1
  [VVMC_ACCLowSpdTqCtrl_flg] -> NOT8/1
  Constant120/1 -> Relational Operator54/2
  Relational Operator54/1 -> AND5/1
  [VVMC_ACCDeltaAccel_mps2] -> Relational Operator54/1
  [VVMC_ACCDeltaAccel_mps2] -> Relational Operator58/1
  Logical Operator9/1 -> SR_Latch4/2
  OR7/1 -> SR_Latch5/2
  [VVMC_OriADASWhlTq_Nm] -> Triggered Subsystem1/1(In1)
  Switch36/1 -> Add5/1
  [VVMC_ACCVehHoldReqRaw_flg] -> AND6/2
  Logical Operator6/1 -> SR_Latch3/1
  [VVMC_AccelTurnHold_flg] -> AND29/1
  Constant74/1 -> Switch5/3
  Add22/1 -> Saturation Dynamic2/1
  Switch39/1 -> Switch7/3  "VVMC_ADASWhlTqCalVehHold_Nm"
  Constant65/1 -> Max5/2
  [VVMC_LastADASWhlTqCal_Nm] -> Add19/1
  Saturation Dynamic2/1 -> Max5/1
  Add19/1 -> Saturation Dynamic2/3
  Max9/1 -> Saturation Dynamic2/2
  [task_time_s] -> Divide7/2
  AND7/1 -> Switch25/2
  AND6/1 -> SR_Latch2/1
  Constant121/1 -> Relational Operator59/2
  Constant106/1 -> Relational Operator13/2
  Constant107/1 -> Relational Operator52/2
  [VVMC_LastADASWhlTqCal_Nm] -> u2 > 0 (4)/1, Abs/1
  Unit Delay4/1 -> NOT4/1
  Constant111/1 -> NOT10/1
  [VVMC_EstSlope_Deg] -> MVMC_VehHoldTqIncGain_Y_Nm/1
  SR_Latch2/1 -> [VVMC_HoldNoMCP_flg]  "VVMC_HoldNoMCP_flg"
  Cast To Single3/1 -> Saturation Dynamic3/2
  Switch28/1 -> Switch39/3
  NOT10/1 -> AND7/2
  [VTQD_CreepBaseTqD_Nm] -> Max9/1
  Constant108/1 -> Relational Operator53/2
  NOT6/1 -> OR4/1
  Relational Operator37/1 -> Logical Operator7/2
  Max5/1 -> Switch41/3  "VVMC_ADASWhlTqVehHoldBfrSS_Nm"
  Constant82/1 -> Relational Operator36/2
  AND29/1 -> Switch39/2
  [VVMC_ACCVehHoldReqRaw_flg] -> NOT6/1
  Constant122/1 -> Add19/2
  Max6/1 -> Saturation Dynamic3/3
  MVMC_VehHoldTqIncGain_Y_Nm/1 -> Divide8/1, Switch31/1
  AND12/1 -> u2 > 0 (3)/2
  [VINP_MCPressure_bar] -> Relational Operator52/1
  [VVMC_EstSlope_Deg] -> Equal4/1
  [VVMC_HoldNoMCP_flg] -> Switch31/2
  Constant33/1 -> Switch31/3
  Divide4/1 -> Relational Operator59/1, Switch25/1
  Add16/1 -> Divide4/1
  Relational Operator51/1 -> Switch28/2
  Constant104/1 -> Equal4/2
  Switch30/1 -> Switch28/1
  Constant32/1 -> Divide4/2
  Switch7/1 -> Switch11/3
  Relational Operator13/1 -> AND6/3
  Switch25/1 -> Add17/2
  Switch41/1 -> Switch28/3  "VVMC_ADASWhlTqCalVehHoldPosTq_Nm"
  Add17/1 -> Max9/2
  Switch31/1 -> Switch25/3
  [VINP_ESCADASSta_enum] -> Equal10/1
  Unit Delay12/1 -> Add16/2
  [VINP_MCPressure_bar] -> Unit Delay12/1, Add16/1
  [VVMC_LastADASWhlTqCal_Nm] -> Add17/1
  Constant61/1 -> Relational Operator19/2
  Relational Operator35/1 -> Logical Operator6/4
  Divide8/1 -> Add22/1
  NOT4/1 -> OR6/1
  Constant167/1 -> Divide7/1
  Max8/1 -> Switch41/1
  [VVMC_ADASACCSta_enum] -> Relational Operator73/1
  Constant17/1 -> Relational Operator73/2
  Constant156/1 -> Switch39/1
  [VVMC_LastADASWhlTqCal_Nm] -> Add21/1
  Divide7/1 -> Add21/2
  Add21/1 -> Max8/1
  Relational Operator34/1 -> Logical Operator6/5
  Constant102/1 -> Switch30/3
  Constant168/1 -> Max8/2
  [VVMC_ADASActive_flg] -> NOT7/1
  [VVMC_LastADASWhlTqCal_Nm] -> Add22/2
  Constant11/1 -> Max6/1
  Switch17/1 -> Relational Operator51/1, Switch30/1, Switch7/1, Switch11/1
  Switch5/1 -> Cast To Single3/1
  u2 > 0 (3)/1 -> Switch5/1
  InitialCondition: 1/1 -> [VVMC_LastADASWhlTqCal_Nm]  "VVMC_LastADASWhlTqCal_Nm"
  [VVMC_ACCPedalOvrd_flg] -> Unit Delay4/1
  Constant90/1 -> Relational Operator39/2
  [VINP_MCPressure_bar] -> Relational Operator53/1
  [VVMC_TotalAvailBrkRgnTq_Nm] -> Max6/2
  Relational Operator38/1 -> Logical Operator7/1
  Logical Operator7/1 -> SR_Latch3/2
  Relational Operator18/1 -> u2 > 0 (4)/2
  u2 > 0 (4)/1 -> u2 > 0 (3)/1  "VVMC_ADASWhlTqCalAftSafety_Nm"
  NOT7/1 -> Logical Operator7/3
  Equal4/1 -> AND29/2
  OR6/1 -> OR5/2
  OR5/1 -> Switch5/2
  Abs/1 -> Relational Operator18/1
  [VINP_VehSpeed_kph] -> Relational Operator34/1
  [VVMC_ActACCRequiredAccel_mps2] -> Unit Delay8/1
  SR_Latch3/1 -> [VVMC_RgnProhibited_flg]  "VVMC_RgnProhibited_flg"
  Saturation Dynamic3/1 -> [VVMC_ADASWhlTqCal_Nm], InitialCondition: 1/1  "VVMC_ADASWhlTqCal_Nm"
  [VVMC_LastADASWhlTqCal_Nm] -> Relational Operator39/1
  Relational Operator36/1 -> Logical Operator6/3
  [VVMC_MCPreBaseTqEn_flg] -> Switch11/2
  [VVMC_FeatArbitrFinal_enum] -> Relational Operator19/1
  [VVMC_SafetyCtrl_flg] -> AND12/3
  OR4/1 -> SR_Latch2/2
  Constant80/1 -> Relational Operator34/2
  Constant81/1 -> Relational Operator35/2
  [VVMC_ActACCRequiredAccel_mps2] -> Relational Operator35/1
  Constant88/1 -> Relational Operator38/2
  Constant87/1 -> Relational Operator37/2
  Constant10/1 -> Saturation Dynamic3/1
  NOT3/1 -> Switch7/2
  Switch11/1 -> Abs1/1, u2 > 0 (4)/3, u2 > 0 (3)/3
  Relational Operator19/1 -> AND12/2
  Constant166/1 -> Equal10/2
  Abs1/1 -> Relational Operator18/2
  [VINP_VehSpeed_kph] -> Relational Operator38/1
  Equal10/1 -> Switch41/2
  Relational Operator59/1 -> AND7/1
  Relational Operator73/1 -> OR6/2
  [VVMC_ACCLowSpdFollowESCTq_flg] -> OR8/1
  Constant103/1 -> Relational Operator51/2
  Relational Operator53/1 -> OR4/2
  Constant30/1 -> AND12/1
  Relational Operator52/1 -> AND6/1
  [VVMC_ActACCRequiredAccel_mps2] -> Relational Operator37/1
  [VVMC_ACCVehHoldReqRaw_flg] -> NOT3/1
  Unit Delay8/1 -> Relational Operator36/1
  Constant44/1 -> Relational Operator61/2
  [VINP_VehSpeed_kph] -> Relational Operator61/1
  OR8/1 -> Switch30/2
  [VVMC_LastADASWhlTqCal_Nm] -> Relational Operator13/1
  Relational Operator39/1 -> Logical Operator6/2
  Relational Operator61/1 -> OR8/2
  [VVMC_ADASActive_flg] -> OR5/1
  Constant133/1 -> Divide8/2
  [VVMC_ACCPedalOvrd_flg] -> Unit Delay13/1
  Unit Delay13/1 -> Detect Decrease1/1
  Detect Decrease1/1 -> Switch36/2
  Constant86/1 -> Add23/2
  Constant94/1 -> Min5/2
  Add23/1 -> Min5/1
  NOT8/1 -> OR7/2
  Min5/1 -> Switch36/1
  VVMC_OVRD2ActRampActive_flg/1 -> [VVMC_OVRD2ActRampActive_flg]
  VINP_ACCRequiredAccel_mps2/1 -> [VINP_ACCRequiredAccel_mps2]
  [VVMC_OVRD2ActRampActive_flg] -> AND9/1
  [VINP_ACCRequiredAccel_mps2] -> Relational Operator1/1
  Constant18/1 -> Relational Operator1/2
  Relational Operator1/1 -> AND9/2
  Constant23/1 -> AND9/3
  [VVMC_LastADASWhlTqCal_Nm] -> Relational Operator27/1
  Constant24/1 -> Relational Operator27/2
  Relational Operator27/1 -> AND9/4
  AND9/1 -> [VVMC_OVRDAccCtrl_flg], Switch9/2  "VVMC_OVRDAccCtrl_flg"
  [VVMC_ActACCRequiredAccel_mps2] -> Switch9/3
  [VINP_ACCRequiredAccel_mps2] -> Switch9/1
  [VVMC_OVRDAccCtrl_flg] -> Switch26/2
  MVMC_ACCDeltaTqIGain4OVRD_Z_Nm/1 -> Switch26/1  "VVMC_ACCDeltaTqIGain4OVRD_Nm"
  [VINP_VehSpeed_kph] -> MVMC_ACCDeltaTqIGain4OVRD_Z_Nm/2
  Switch26/1 -> Switch34/3
  [VVMC_DISCDeltaTqIGain_Nm] -> Switch33/1
  Equal12/1 -> AND18/2
  Equal11/1 -> AND18/1
  Constant68/1 -> Equal11/2
  Constant71/1 -> Equal12/2
  [VVMC_ActACCRequiredAccel_mps2] -> Equal12/1
  [VVMC_LongAcc_Gps] -> Equal11/1
  Switch40/1 -> Switch34/1
  AND18/1 -> Switch40/2
  [VVMC_ActAccDev_mps2] -> MVMC_ADSPosGFBDeltaTq_Z_Nm1/1
  [VINP_VehSpeed_kph] -> MVMC_ADSPosGFBDeltaTq_Z_Nm1/2
  MVMC_ADSPosGFBDeltaTq_Z_Nm1/1 -> Switch40/3  "VVMC_ADSPosGFBPCTDeltaTq_Nm"
  [VINP_SWCType_enum] -> Relational Operator56/1
  " 2"/1 -> Relational Operator56/2
  Relational Operator56/1 -> Switch2/2
  [VTQD_SWC2ResUpSta_flg] -> Switch2/1
  VTQD_SWC1ResUpSta_flg/1 -> [VTQD_SWC1ResUpSta_flg]
  [VTQD_SWC1ResUpSta_flg] -> Switch2/3
  VINP_SWCType_enum/1 -> [VINP_SWCType_enum]
  [VTQD_SWC1ResUpSta_flg] -> Switch32/3
  [VTQD_SWC2ResUpSta_flg] -> Switch32/1
  Relational Operator57/1 -> Switch32/2
  " 1"/1 -> Relational Operator57/2
  [VINP_SWCType_enum] -> Relational Operator57/1
  [VVMC_ADASActive_flg] -> Logical Operator6/1
  [VVMC_ADASActive_flg] -> Logical Operator8/1

== system vmc/VMC/VMC/APS function/CAAS HandShake ==
  VINP_VehSpeed_kph : Inport
  VVMC_ADASActive_flg : Inport  Port=2
  VVMC_CruzActive_flg : Inport  Port=3
  task_time_s : Inport  Port=4
  VINP_CAASVMCReqA_flg : Inport  Port=5
  AND : Logic  Inputs=3  AllPortsSameDT=off  OutDataTypeStr=boolean
  AND1 : Logic  AllPortsSameDT=off  OutDataTypeStr=boolean
  Constant1 : Constant  Value=KVMC_CAASCtrlAllowTime_s
  Constant11 : Constant  Value=KVMC_CAASEnVehSpd_kph
  Constant2 : Constant  Value=KVMC_CAASVMCReqA_flg_ovrdflg
  Constant3 : Constant  Value=KVMC_CAASVMCReqA_flg_ovrdval
  DelayEnable : hcu_lib/Basic_Blocks/DelayEnable
  NOT : Logic  Operator=NOT  AllPortsSameDT=off  OutDataTypeStr=boolean
  NOT1 : Logic  Operator=NOT  AllPortsSameDT=off  OutDataTypeStr=boolean
  Relational Operator : RelationalOperator  Operator=<=  OutDataTypeStr=boolean  RndMeth=Simplest
  Switch : Switch  Criteria=u2 > Threshold
  VVMC_CAASCtrlAvail_flg : Outport
  VVMC_CAASActive_flg : Outport  Port=2
  wires:
  Relational Operator/1 -> AND/1
  VVMC_ADASActive_flg/1 -> [VVMC_ADASActive_flg]
  VINP_VehSpeed_kph/1 -> [VINP_VehSpeed_kph]
  AND/1 -> DelayEnable/1
  Constant1/1 -> DelayEnable/2
  task_time_s/1 -> [task_time_s]
  [VINP_VehSpeed_kph] -> Relational Operator/1
  [VVMC_CruzActive_flg] -> NOT1/1
  VVMC_CruzActive_flg/1 -> [VVMC_CruzActive_flg]
  Constant11/1 -> Relational Operator/2
  DelayEnable/1 -> [VVMC_CAASCtrlAvail_flg]  "VVMC_CAASCtrlAvail_flg"
  [task_time_s] -> DelayEnable/3
  NOT1/1 -> AND/3
  NOT/1 -> AND/2
  [VVMC_ADASActive_flg] -> NOT/1
  [VVMC_CAASCtrlAvail_flg] -> VVMC_CAASCtrlAvail_flg/1
  [VVMC_CAASCtrlAvail_flg] -> AND1/1
  VINP_CAASVMCReqA_flg/1 -> [VINP_CAASVMCReqA_flg]
  AND1/1 -> [VVMC_CAASActive_flg]  "VVMC_CAASActive_flg"
  [VVMC_CAASActive_flg] -> VVMC_CAASActive_flg/1
  [VINP_CAASVMCReqA_flg] -> Switch/3
  Switch/1 -> AND1/2
  Constant3/1 -> Switch/1
  Constant2/1 -> Switch/2

== system vmc/VMC/VMC/APS function/Command Determination1 ==
  VVMC_APSActive_flg : Inport
  VINP_APSStaSys_enum : Inport  Port=2
  VINP_APSShiftPosnReq_enum : Inport  Port=3
  VINP_APSSpeedCMD_kph : Inport  Port=4
  AND : Logic  AllPortsSameDT=off  OutDataTypeStr=boolean
  Constant : Constant  Value=ENUM_APSSYSTEMSTA_ACTIVE
  Constant1 : Constant  Value=ENUM_APSSYSTEMSTA_REMOTEACTIVE
  Constant2 : Constant  Value=ZERO_FLOAT
  Constant3 : Constant  Value=ENUM_APSSHIFTPOSNREQ_PARK
  Equal : RelationalOperator  Operator===  OutDataTypeStr=boolean  RndMeth=Simplest
  Equal1 : RelationalOperator  Operator===  OutDataTypeStr=boolean  RndMeth=Simplest
  OR : Logic  Operator=OR  AllPortsSameDT=off  OutDataTypeStr=boolean
  Switch : Switch  Criteria=u2 > Threshold
  Switch1 : Switch  Criteria=u2 > Threshold
  VVMC_APSSpeedCMD_kph : Outport
  VVMC_APSShiftPosnReq_enum : Outport  Port=2
  wires:
  [VVMC_APSEnCMD_flg] -> Switch1/2
  [VINP_APSShiftPosnReq_enum] -> Switch1/1
  Constant3/1 -> Switch1/3
  Switch1/1 -> VVMC_APSShiftPosnReq_enum/1  "VVMC_APSShiftPosnReq_enum"
  Switch/1 -> VVMC_APSSpeedCMD_kph/1  "VVMC_APSSpeedCMD_kph"
  Constant2/1 -> Switch/3
  [VINP_APSSpeedCMD_kph] -> Switch/1
  [VVMC_APSEnCMD_flg] -> Switch/2
  AND/1 -> [VVMC_APSEnCMD_flg]  "VVMC_APSEnCMD_flg"
  OR/1 -> AND/2
  [VVMC_APSActive_flg] -> AND/1
  Equal1/1 -> OR/2
  Equal/1 -> OR/1
  [VINP_APSStaSys_enum] -> Equal1/1
  Constant1/1 -> Equal1/2
  Constant/1 -> Equal/2
  [VINP_APSStaSys_enum] -> Equal/1
  VINP_APSSpeedCMD_kph/1 -> [VINP_APSSpeedCMD_kph]
  VINP_APSShiftPosnReq_enum/1 -> [VINP_APSShiftPosnReq_enum]
  VINP_APSStaSys_enum/1 -> [VINP_APSStaSys_enum]
  VVMC_APSActive_flg/1 -> [VVMC_APSActive_flg]

== system vmc/VMC/VMC/APS function/Hand Shake ==
  task_time_s : Inport
  VTQD_ExternalTqAllow_flg : Inport  Port=2
  VTQD_ExtShiftAllow_flg : Inport  Port=3
  VINP_APSVMCReqA_flg : Inport  Port=4
  VINP_APSStaSys_enum : Inport  Port=5
  VTQD_ExtDoorAllow_flg : Inport  Port=6
  VTQD_GearActualPosn_enum : Inport  Port=7
  VDDM_VCURAPSErrLv2_flg : Inport  Port=8
  VDDM_VCURAPSErrLv3_flg : Inport  Port=9
  VTQD_EPBCarWashMode_flg : Inport  Port=10
  AND : Logic  Inputs=4  AllPortsSameDT=off  OutDataTypeStr=boolean
  AND1 : Logic  Inputs=3  AllPortsSameDT=off  OutDataTypeStr=boolean
  AND2 : Logic  Inputs=4  AllPortsSameDT=off  OutDataTypeStr=boolean
  Constant : Constant  Value=KVMC_ExternalTqAllowTime_s
  Constant1 : Constant  Value=KVMC_ExternalShiftAllowTime_s
  Constant2 : Constant  Value=ENUM_APSSYSTEMSTA_ACTIVE
  Constant3 : Constant  Value=ENUM_APSSYSTEMSTA_REMOTEACTIVE
  Constant4 : Constant  Value=KVMC_ExternalDoorAllowTime_s
  Delay : Delay  DelayLength=1
  Delay1 : Delay  DelayLength=1
  DelayEnable : hcu_lib/Basic_Blocks/DelayEnable
  DelayEnable1 : hcu_lib/Basic_Blocks/DelayEnable
  DelayEnable2 : hcu_lib/Basic_Blocks/DelayEnable
  Detect Decrease : simulink/Logic and Bit Operations/Detect Decrease  vinit=0.0  OutDataTypeStr=boolean
  Equal : RelationalOperator  Operator===  OutDataTypeStr=boolean  RndMeth=Simplest
  Equal1 : RelationalOperator  Operator===  OutDataTypeStr=boolean  RndMeth=Simplest
  Logical Operator : Logic  Operator=NOT  AllPortsSameDT=off  OutDataTypeStr=boolean
  Logical Operator1 : Logic  Operator=NOT  AllPortsSameDT=off  OutDataTypeStr=boolean
  Logical Operator2 : Logic  Operator=NOT  AllPortsSameDT=off  OutDataTypeStr=boolean
  NOT : Logic  Operator=NOT  AllPortsSameDT=off  OutDataTypeStr=boolean
  OR : Logic  Operator=OR  AllPortsSameDT=off  OutDataTypeStr=boolean
  SR_Latch : hcu_lib/Basic_Blocks/SR_Latch
  VVMC_APSCtrlAvail_flg : Outport
  VVMC_APSActive_flg : Outport  Port=2
  wires:
  VINP_APSVMCReqA_flg/1 -> [VINP_APSVMCReqA_flg]
  VTQD_ExtShiftAllow_flg/1 -> [VTQD_ExtShiftAllow_flg]
  [task_time_s] -> DelayEnable1/3
  Constant1/1 -> DelayEnable1/2
  DelayEnable1/1 -> [VVMC_APSShiftCtrlAllow_flg]  "VVMC_APSShiftCtrlAllow_flg"
  [VTQD_ExtShiftAllow_flg] -> DelayEnable1/1
  [VTQD_ExternalTqAllow_flg] -> DelayEnable/1
  VTQD_ExternalTqAllow_flg/1 -> [VTQD_ExternalTqAllow_flg]
  task_time_s/1 -> [task_time_s]
  DelayEnable/1 -> [VVMC_APSTqCtrlAllow_flg]  "VVMC_APSTqCtrlAllow_flg"
  Constant/1 -> DelayEnable/2
  [task_time_s] -> DelayEnable/3
  Constant2/1 -> Equal/2
  [VINP_APSStaSys_enum] -> Equal/1
  Equal/1 -> OR/1
  OR/1 -> AND1/3
  [VINP_APSVMCReqA_flg] -> AND1/1
  Constant3/1 -> Equal1/2
  Equal1/1 -> OR/2
  [VINP_APSStaSys_enum] -> Equal1/1
  [VVMC_APSCtrlAvail_flg] -> AND1/2
  AND1/1 -> [VVMC_APSActive_flg], VVMC_APSActive_flg/1  "VVMC_APSActive_flg"
  VINP_APSStaSys_enum/1 -> [VINP_APSStaSys_enum]
  VTQD_ExtDoorAllow_flg/1 -> [VTQD_ExtDoorAllow_flg]
  Constant4/1 -> DelayEnable2/2
  DelayEnable2/1 -> [VVMC_APSDoorCtrlAllow_flg]  "VVMC_APSDoorCtrlAllow_flg"
  [task_time_s] -> DelayEnable2/3
  [VTQD_ExtDoorAllow_flg] -> DelayEnable2/1
  AND/1 -> [VVMC_APSCtrlAvail_flg], VVMC_APSCtrlAvail_flg/1  "VVMC_APSCtrlAvail_flg"
  [VVMC_APSTqCtrlAllow_flg] -> AND/1
  VDDM_VCURAPSErrLv3_flg/1 -> [VDDM_VCURAPSErrLv3_flg]
  VDDM_VCURAPSErrLv2_flg/1 -> [VDDM_VCURAPSErrLv2_flg]
  VTQD_GearActualPosn_enum/1 -> [VTQD_GearActualPosn_enum]
  VTQD_EPBCarWashMode_flg/1 -> [VTQD_EPBCarWashMode_flg]
  SR_Latch/1 -> AND/2
  [VVMC_APSDoorCtrlAllow_flg] -> AND2/2
  Logical Operator/1 -> AND2/3
  [VVMC_APSShiftCtrlAllow_flg] -> AND2/1
  [VTQD_EPBCarWashMode_flg] -> Logical Operator1/1
  NOT/1 -> AND2/4
  [VDDM_VCURAPSErrLv3_flg] -> Logical Operator2/1
  Delay1/1 -> Detect Decrease/1
  AND2/1 -> SR_Latch/1
  [VDDM_VCURAPSErrLv2_flg] -> Logical Operator/1
  [VVMC_APSActive_flg] -> Delay1/1
  Logical Operator2/1 -> AND/3
  Detect Decrease/1 -> SR_Latch/2
  Logical Operator1/1 -> AND/4
  Delay/1 -> NOT/1
  [VVMC_APSActive_flg] -> Delay/1
